simulink model "h2_containment_static_3d"  (R2022b)
settings: Solver=FixedStepAuto  StartTime=0.0  StopTime=15  FixedStep=0.01  RelTol=1e-3
values from neighbouring files (symbols this model uses):
  A = [0, 0,-1 ;0 0 2; 1 0  -1.5]    [containment_staic_3d.m]    (also in containment_staic_3d_paper.m)
  Af = kron(IM,A)    [containment_staic_3d.m]    (also in containment_staic_3d_paper.m)
  Al = kron(Inm,A)    [containment_staic_3d.m]    (also in containment_staic_3d_paper.m)
  Bf = kron(IM,B)    [containment_staic_3d.m]    (also in containment_staic_3d_paper.m)
  Cd = kron(IM,C)+kron(L1,D*K)    [containment_staic_3d.m]    (also in containment_staic_3d_paper.m)
  Ef = kron(IM,E)    [containment_staic_3d.m]    (also in containment_staic_3d_paper.m)
  Kk = kron(IM,K)    [containment_staic_3d.m]    (also in containment_staic_3d_paper.m)
  Lk1 = kron(L1,eye(3))    [containment_staic_3d.m]    (also in containment_staic_3d_paper.m)
  Lk2 = kron(L2,eye(3))    [containment_staic_3d.m]    (also in containment_staic_3d_paper.m)
  xf = xint(1:18)'    [containment_staic_3d.m]    (also in containment_staic_3d_paper.m)
  Xint = kron(L1,eye(3))*xf+kron(L2,eye(3))*xl    [containment_staic_3d.m]    (also in containment_staic_3d_paper.m)
  xl = xint(19:27)'    [containment_staic_3d.m]    (also in containment_staic_3d_paper.m)
settings Model: Creator=lenovo  LastModifiedBy=herrg
settings SolverCC: AlgebraicLoopSolver=TrustRegion
settings DebuggingCC: UnconnectedInputMsg=warning  UnconnectedOutputMsg=warning  UnconnectedLineMsg=warning  SFMachineParentedDataDiag=warning
settings ModelReferenceCC: EnableRefExpFcnMdlSchedulingChecks=on
settings RTWCC: DLArmComputeVersion=19.05

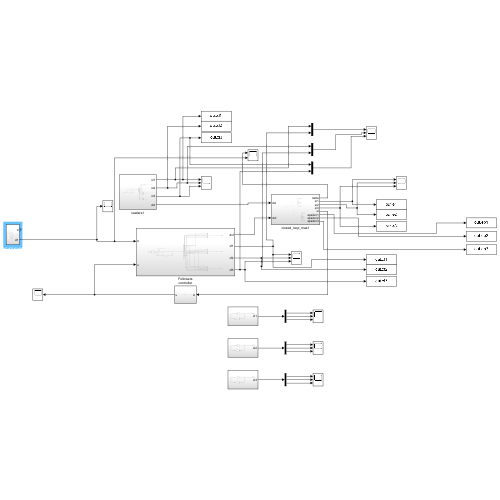
[thumbnail: Simulink's stored preview of the top-level diagram]
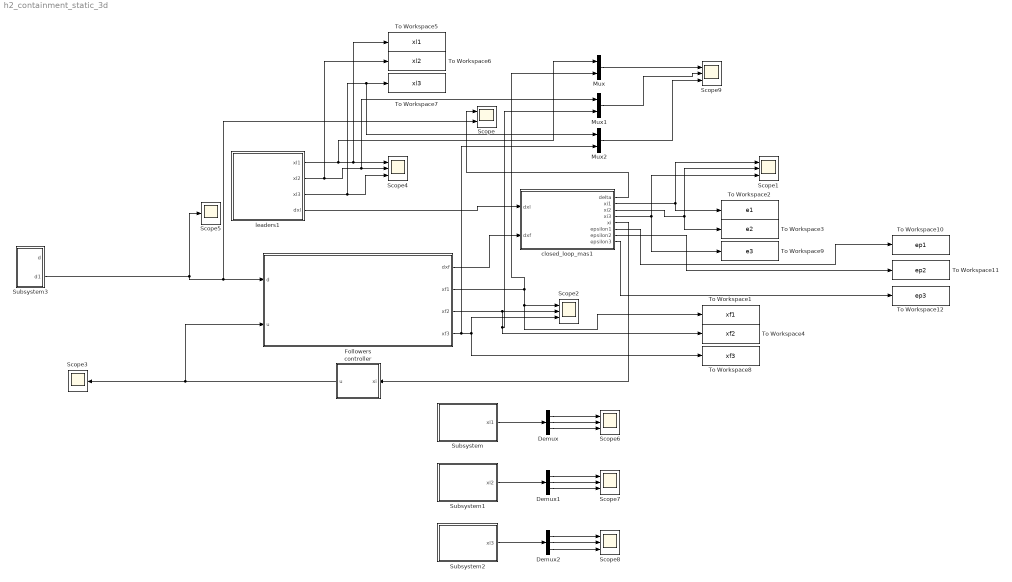
== system h2_containment_static_3d ==
  Demux : Demux  Outputs=3
  Demux1 : Demux  Outputs=3
  Demux2 : Demux  Outputs=3
  Followers : Subsystem
  Mux : Mux  Inputs=2
  Mux1 : Mux  Inputs=2
  Mux2 : Mux  Inputs=2
  Scope : Scope  NumInputPorts=2
  Scope{1..2,4,6..9} (7 alike) : Scope  NumInputPorts=3
  Scope3 : Scope
  Scope5 : Scope
  Subsystem : Subsystem
  Subsystem1 : Subsystem
  Subsystem2 : Subsystem
  Subsystem3 : Subsystem
  To Workspace1 : ToWorkspace  VariableName=xf1  SampleTime=-1
  To Workspace10 : ToWorkspace  VariableName=ep1  SampleTime=-1
  To Workspace11 : ToWorkspace  VariableName=ep2  SampleTime=-1
  To Workspace12 : ToWorkspace  VariableName=ep3  SampleTime=-1
  To Workspace2 : ToWorkspace  VariableName=e1  SampleTime=-1
  To Workspace3 : ToWorkspace  VariableName=e2  SampleTime=-1
  To Workspace4 : ToWorkspace  VariableName=xf2  SampleTime=-1
  To Workspace5 : ToWorkspace  VariableName=xl1  SampleTime=-1
  To Workspace6 : ToWorkspace  VariableName=xl2  SampleTime=-1
  To Workspace7 : ToWorkspace  VariableName=xl3  SampleTime=-1
  To Workspace8 : ToWorkspace  VariableName=xf3  SampleTime=-1
  To Workspace9 : ToWorkspace  VariableName=e3  SampleTime=-1
  closed_loop_mas1 : Subsystem
  controller : Subsystem
  leaders1 : Subsystem
  wires:
  leaders1/2(xl2) -> Scope4/2, Mux1/1, To Workspace6/1
  closed_loop_mas1/1(delta) -> Scope/1
  Followers/3(xf2) -> Scope2/2, Mux1/2, To Workspace4/1
  Followers/2(xf1) -> To Workspace1/1, Scope2/1, Mux/2
  closed_loop_mas1/5(xi) -> controller/1(xi)
  closed_loop_mas1/3(xi2) -> Scope1/2, To Workspace3/1
  closed_loop_mas1/2(xi1) -> To Workspace2/1, Scope1/1
  Demux1/1 -> Scope7/1
  Subsystem1/1(xl2) -> Demux1/1
  Demux1/2 -> Scope7/2
  leaders1/4(dxl) -> closed_loop_mas1/1(dxl)
  Followers/1(dxf) -> closed_loop_mas1/2(dxf)
  controller/1(u) -> Followers/2(u), Scope3/1
  Demux/2 -> Scope6/2
  Mux1/1 -> Scope9/2
  leaders1/1(xl1) -> Mux/1, To Workspace5/1, Scope4/1
  Demux/1 -> Scope6/1
  Mux/1 -> Scope9/1
  Demux2/2 -> Scope8/2
  Demux2/1 -> Scope8/1
  Subsystem/1(xl1) -> Demux/1
  Subsystem2/1(xl3) -> Demux2/1
  Demux/3 -> Scope6/3
  Demux1/3 -> Scope7/3
  Demux2/3 -> Scope8/3
  leaders1/3(xl3) -> Mux2/1, To Workspace7/1, Scope4/3
  Followers/4(xf3) -> Mux2/2, To Workspace8/1, Scope2/3
  closed_loop_mas1/4(xi3) -> To Workspace9/1, Scope1/3
  Mux2/1 -> Scope9/3
  closed_loop_mas1/6(epsilon1) -> To Workspace10/1
  closed_loop_mas1/7(epsilon2) -> To Workspace11/1
  closed_loop_mas1/8(epsilon3) -> To Workspace12/1
  Subsystem3/2(d1) -> Scope5/1, Scope/2, Followers/1(d)

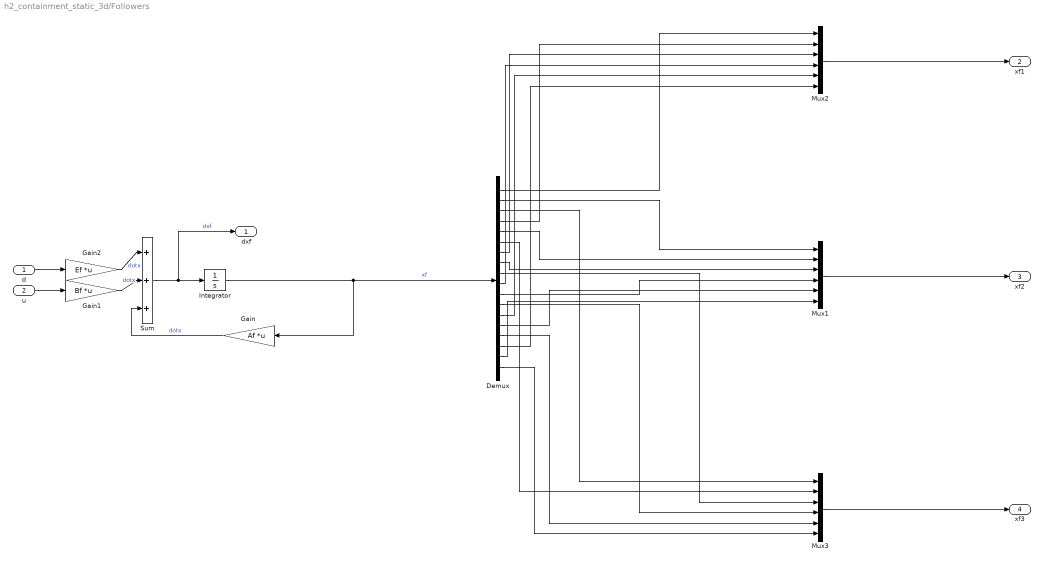
== system h2_containment_static_3d/Followers ==
  d : Inport
  u : Inport  Port=2
  Demux : Demux  Outputs=18
  Gain : Gain  Gain=Af  Multiplication=Matrix(K*u) (u vector)
  Gain1 : Gain  Gain=Bf  Multiplication=Matrix(K*u) (u vector)
  Gain2 : Gain  Gain=Ef  Multiplication=Matrix(K*u) (u vector)
  Integrator : Integrator  InitialCondition=xf
  Mux1 : Mux  Inputs=6
  Mux2 : Mux  Inputs=6
  Mux3 : Mux  Inputs=6
  Sum : Sum  Inputs=|+++
  dxf : Outport
  xf1 : Outport  Port=2
  xf2 : Outport  Port=3
  xf3 : Outport  Port=4
  wires:
  Gain/1 -> Sum/3  "dotx"
  u/1 -> Gain1/1
  d/1 -> Gain2/1
  Gain1/1 -> Sum/2  "dotx"
  Gain2/1 -> Sum/1  "dotx"
  Sum/1 -> dxf/1, Integrator/1  "dxf"
  Integrator/1 -> Gain/1, Demux/1  "xf"
  Mux2/1 -> xf1/1
  Mux1/1 -> xf2/1
  Mux3/1 -> xf3/1
  Demux/1 -> Mux2/1
  Demux/2 -> Mux1/1
  Demux/3 -> Mux3/1
  Demux/4 -> Mux2/2
  Demux/5 -> Mux1/2
  Demux/6 -> Mux3/2
  Demux/7 -> Mux2/3
  Demux/8 -> Mux1/3
  Demux/9 -> Mux3/3
  Demux/10 -> Mux2/4
  Demux/11 -> Mux1/4
  Demux/12 -> Mux3/4
  Demux/13 -> Mux2/5
  Demux/14 -> Mux1/5
  Demux/15 -> Mux3/5
  Demux/16 -> Mux2/6
  Demux/17 -> Mux1/6
  Demux/18 -> Mux3/6

== system h2_containment_static_3d/Subsystem ==
  Gain2 : Gain  Gain=A  Multiplication=Matrix(K*u) (u vector)
  Integrator : Integrator  InitialCondition=xl(1:3)
  xl1 : Outport
  wires:
  Integrator/1 -> xl1/1, Gain2/1  "x"
  Gain2/1 -> Integrator/1  "dotx"

== system h2_containment_static_3d/Subsystem1 ==
  Gain2 : Gain  Gain=A  Multiplication=Matrix(K*u) (u vector)
  Integrator : Integrator  InitialCondition=xl(4:6)
  xl2 : Outport
  wires:
  Integrator/1 -> xl2/1, Gain2/1  "x"
  Gain2/1 -> Integrator/1  "dotx"

== system h2_containment_static_3d/Subsystem2 ==
  Gain2 : Gain  Gain=A  Multiplication=Matrix(K*u) (u vector)
  Integrator : Integrator  InitialCondition=xl(7:9)
  xl3 : Outport
  wires:
  Integrator/1 -> xl3/1, Gain2/1  "x"
  Gain2/1 -> Integrator/1  "dotx"

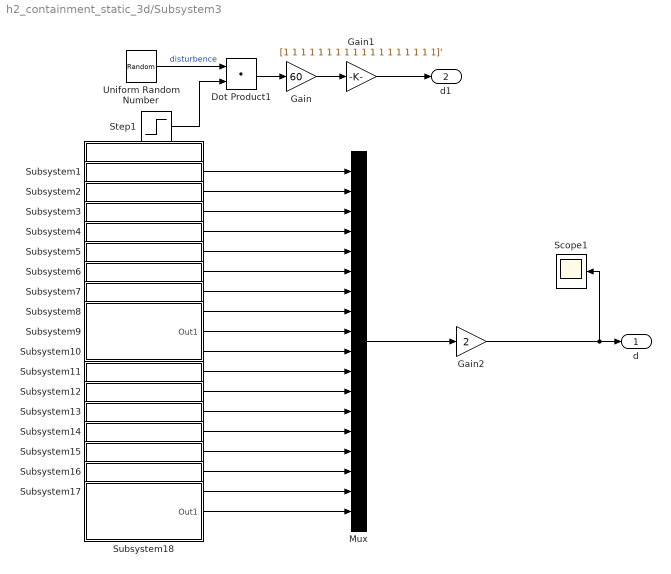
== system h2_containment_static_3d/Subsystem3 ==
  Dot Product1 : DotProduct  OutDataTypeStr=Inherit: Inherit via internal rule
  Gain : Gain  Gain=60
  Gain1 : Gain  Gain=[1 1 1 1 1 1 1 1 1 1 1 1 1 1 1 1 1 1]'
  Gain2 : Gain  Gain=2
  Mux : Mux  Inputs=18
  Scope1 : Scope
  Step1 : Step  Time=1000  Before=1  After=0  SampleTime=0
  Subsystem1 : Subsystem
  Subsystem10 : Subsystem
  Subsystem11 : Subsystem
  Subsystem12 : Subsystem
  Subsystem13 : Subsystem
  Subsystem14 : Subsystem
  Subsystem15 : Subsystem
  Subsystem16 : Subsystem
  Subsystem17 : Subsystem
  Subsystem18 : Subsystem
  Subsystem2 : Subsystem
  Subsystem3 : Subsystem
  Subsystem4 : Subsystem
  Subsystem5 : Subsystem
  Subsystem6 : Subsystem
  Subsystem7 : Subsystem
  Subsystem8 : Subsystem
  Subsystem9 : Subsystem
  Uniform Random Number : UniformRandomNumber  SampleTime=0.1
  d : Outport
  d1 : Outport  Port=2
  wires:
  Gain1/1 -> d1/1
  Gain/1 -> Gain1/1
  Step1/1 -> Dot Product1/2
  Dot Product1/1 -> Gain/1
  Uniform Random Number/1 -> Dot Product1/1  "disturbence"
  Subsystem13/1(Out1) -> Mux/13
  Subsystem11/1(Out1) -> Mux/11
  Subsystem18/1(Out1) -> Mux/18
  Mux/1 -> Gain2/1
  Subsystem9/1(Out1) -> Mux/9
  Subsystem10/1(Out1) -> Mux/10
  Subsystem8/1(Out1) -> Mux/8
  Subsystem15/1(Out1) -> Mux/15
  Subsystem7/1(Out1) -> Mux/7
  Subsystem14/1(Out1) -> Mux/14
  Subsystem17/1(Out1) -> Mux/17
  Subsystem16/1(Out1) -> Mux/16
  Subsystem4/1(Out1) -> Mux/4
  Subsystem3/1(Out1) -> Mux/3
  Subsystem1/1(Out1) -> Mux/1
  Subsystem2/1(Out1) -> Mux/2
  Subsystem12/1(Out1) -> Mux/12
  Subsystem6/1(Out1) -> Mux/6
  Subsystem5/1(Out1) -> Mux/5
  Gain2/1 -> Scope1/1, d/1

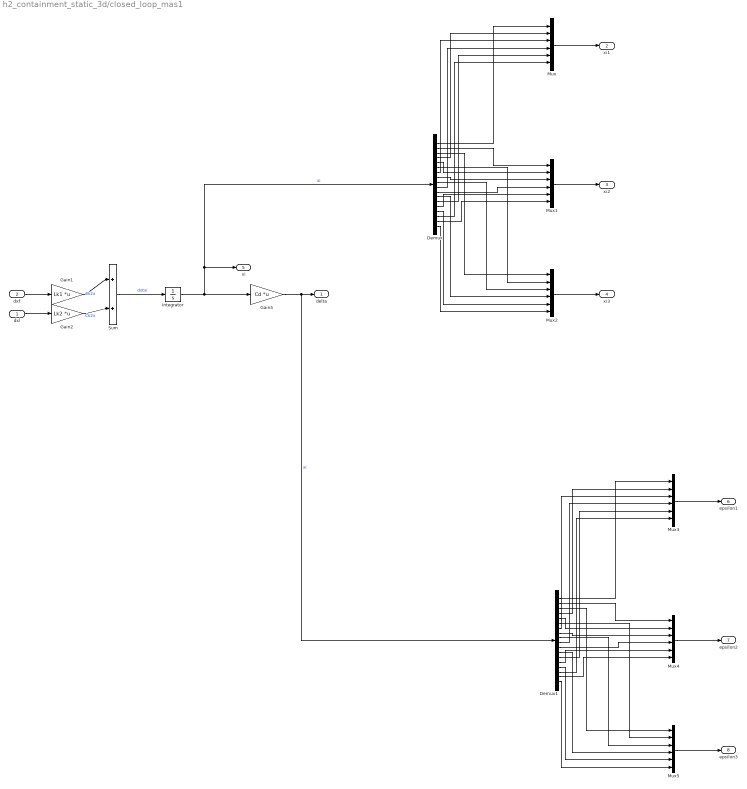
== system h2_containment_static_3d/closed_loop_mas1 ==
  dxl : Inport
  dxf : Inport  Port=2
  Demux : Demux  Outputs=18
  Demux1 : Demux  Outputs=18
  Gain1 : Gain  Gain=Lk1  Multiplication=Matrix(K*u) (u vector)
  Gain2 : Gain  Gain=Lk2  Multiplication=Matrix(K*u) (u vector)
  Gain5 : Gain  Gain=Cd  Multiplication=Matrix(K*u) (u vector)
  Integrator : Integrator  InitialCondition=Xint
  Mux{,1..5} (6 alike) : Mux  Inputs=6
  Sum : Sum  Inputs=|++
  delta : Outport
  xi1 : Outport  Port=2
  xi2 : Outport  Port=3
  xi3 : Outport  Port=4
  xi : Outport  Port=5
  epsilon1 : Outport  Port=6
  epsilon2 : Outport  Port=7
  epsilon3 : Outport  Port=8
  wires:
  Integrator/1 -> Demux/1, xi/1, Gain5/1  "xi"
  Sum/1 -> Integrator/1  "dotxi"
  Mux/1 -> xi1/1
  Mux1/1 -> xi2/1
  dxf/1 -> Gain1/1
  dxl/1 -> Gain2/1
  Gain1/1 -> Sum/1  "Ck2x"
  Gain2/1 -> Sum/2  "Ck2x"
  Mux2/1 -> xi3/1
  Demux/1 -> Mux/1
  Demux/2 -> Mux1/1
  Demux/3 -> Mux2/1
  Demux/4 -> Mux/2
  Demux/5 -> Mux1/2
  Demux/6 -> Mux2/2
  Demux/7 -> Mux/3
  Demux/8 -> Mux1/3
  Demux/9 -> Mux2/3
  Demux/10 -> Mux/4
  Demux/11 -> Mux1/4
  Demux/12 -> Mux2/4
  Demux/13 -> Mux/5
  Demux/14 -> Mux1/5
  Demux/15 -> Mux2/5
  Demux/16 -> Mux/6
  Demux/17 -> Mux1/6
  Demux/18 -> Mux2/6
  Demux1/16 -> Mux3/6
  Demux1/17 -> Mux4/6
  Demux1/4 -> Mux3/2
  Demux1/15 -> Mux5/5
  Demux1/10 -> Mux3/4
  Demux1/14 -> Mux4/5
  Demux1/11 -> Mux4/4
  Demux1/5 -> Mux4/2
  Demux1/7 -> Mux3/3
  Demux1/9 -> Mux5/3
  Demux1/18 -> Mux5/6
  Demux1/13 -> Mux3/5
  Demux1/12 -> Mux5/4
  Demux1/6 -> Mux5/2
  Mux5/1 -> epsilon3/1
  Demux1/2 -> Mux4/1
  Demux1/1 -> Mux3/1
  Demux1/3 -> Mux5/1
  Mux4/1 -> epsilon2/1
  Gain5/1 -> Demux1/1, delta/1  "xi"
  Demux1/8 -> Mux4/3
  Mux3/1 -> epsilon1/1

== system h2_containment_static_3d/controller ==
  xi : Inport
  Gain2 : Gain  Gain=Kk  Multiplication=Matrix(K*u) (u vector)
  u : Outport
  wires:
  Gain2/1 -> u/1
  xi/1 -> Gain2/1

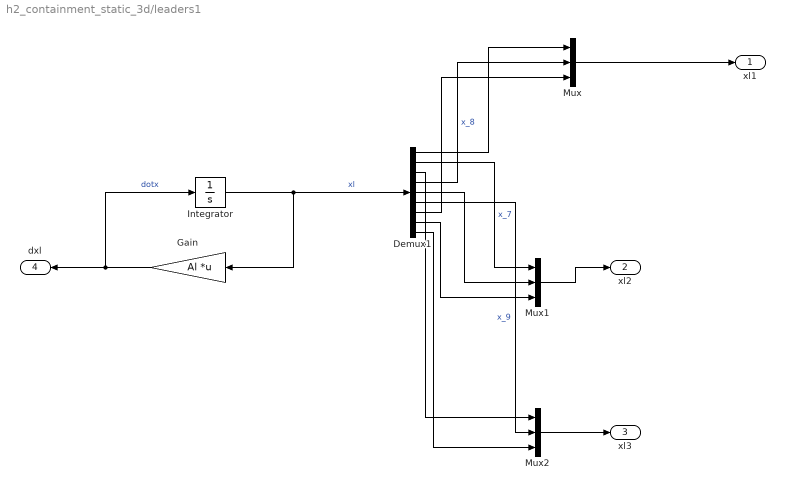
== system h2_containment_static_3d/leaders1 ==
  Demux1 : Demux  Outputs=9
  Gain : Gain  Gain=Al  Multiplication=Matrix(K*u) (u vector)
  Integrator : Integrator  InitialCondition=xl
  Mux : Mux  Inputs=3
  Mux1 : Mux  Inputs=3
  Mux2 : Mux  Inputs=3
  xl1 : Outport
  xl2 : Outport  Port=2
  xl3 : Outport  Port=3
  dxl : Outport  Port=4
  wires:
  Gain/1 -> dxl/1, Integrator/1  "dotx"
  Integrator/1 -> Gain/1, Demux1/1  "xl"
  Mux1/1 -> xl2/1
  Mux/1 -> xl1/1
  Demux1/1 -> Mux/1
  Demux1/4 -> Mux/2  "x_8"
  Demux1/7 -> Mux/3
  Demux1/2 -> Mux1/1  "x_7"
  Demux1/5 -> Mux1/2
  Demux1/8 -> Mux1/3
  Mux2/1 -> xl3/1
  Demux1/3 -> Mux2/1
  Demux1/6 -> Mux2/2  "x_9"
  Demux1/9 -> Mux2/3

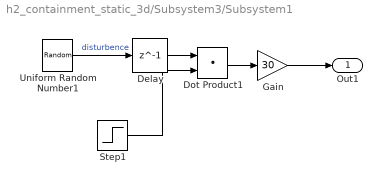
== system h2_containment_static_3d/Subsystem3/Subsystem1 ==
  Delay : Delay  DelayLength=1  SampleTime=0.01
  Dot Product1 : DotProduct  OutDataTypeStr=Inherit: Inherit via internal rule
  Gain : Gain  Gain=30
  Step1 : Step  Time=999  Before=1  After=0  SampleTime=0
  Uniform Random Number1 : UniformRandomNumber  SampleTime=0.1
  Out1 : Outport
  wires:
  Uniform Random Number1/1 -> Delay/1  "disturbence"
  Gain/1 -> Out1/1
  Dot Product1/1 -> Gain/1
  Step1/1 -> Dot Product1/2
  Delay/1 -> Dot Product1/1

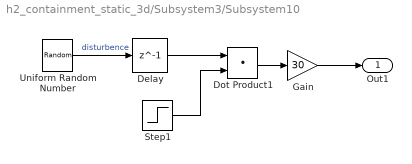
== system h2_containment_static_3d/Subsystem3/Subsystem10 ==
  Delay : Delay  DelayLength=1  SampleTime=0.01
  Dot Product1 : DotProduct  OutDataTypeStr=Inherit: Inherit via internal rule
  Gain : Gain  Gain=30
  Step1 : Step  Time=1000  Before=1  After=0  SampleTime=0
  Uniform Random Number : UniformRandomNumber  SampleTime=0.1
  Out1 : Outport
  wires:
  Uniform Random Number/1 -> Delay/1  "disturbence"
  Step1/1 -> Dot Product1/2
  Gain/1 -> Out1/1
  Dot Product1/1 -> Gain/1
  Delay/1 -> Dot Product1/1

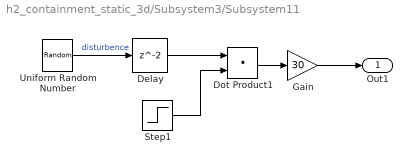
== system h2_containment_static_3d/Subsystem3/Subsystem11 ==
  Delay : Delay  SampleTime=0.01
  Dot Product1 : DotProduct  OutDataTypeStr=Inherit: Inherit via internal rule
  Gain : Gain  Gain=30
  Step1 : Step  Time=1000  Before=1  After=0  SampleTime=0
  Uniform Random Number : UniformRandomNumber  SampleTime=0.1
  Out1 : Outport
  wires:
  Uniform Random Number/1 -> Delay/1  "disturbence"
  Step1/1 -> Dot Product1/2
  Gain/1 -> Out1/1
  Dot Product1/1 -> Gain/1
  Delay/1 -> Dot Product1/1

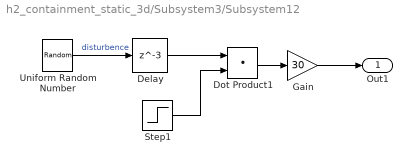
== system h2_containment_static_3d/Subsystem3/Subsystem12 ==
  Delay : Delay  DelayLength=3  SampleTime=0.01
  Dot Product1 : DotProduct  OutDataTypeStr=Inherit: Inherit via internal rule
  Gain : Gain  Gain=30
  Step1 : Step  Time=1000  Before=1  After=0  SampleTime=0
  Uniform Random Number : UniformRandomNumber  SampleTime=0.1
  Out1 : Outport
  wires:
  Uniform Random Number/1 -> Delay/1  "disturbence"
  Step1/1 -> Dot Product1/2
  Gain/1 -> Out1/1
  Dot Product1/1 -> Gain/1
  Delay/1 -> Dot Product1/1

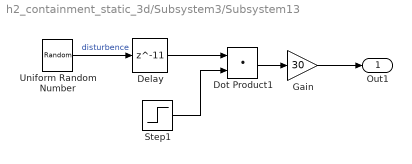
== system h2_containment_static_3d/Subsystem3/Subsystem13 ==
  Delay : Delay  DelayLength=11  SampleTime=0.01
  Dot Product1 : DotProduct  OutDataTypeStr=Inherit: Inherit via internal rule
  Gain : Gain  Gain=30
  Step1 : Step  Time=1000  Before=1  After=0  SampleTime=0
  Uniform Random Number : UniformRandomNumber  SampleTime=0.1
  Out1 : Outport
  wires:
  Uniform Random Number/1 -> Delay/1  "disturbence"
  Step1/1 -> Dot Product1/2
  Gain/1 -> Out1/1
  Dot Product1/1 -> Gain/1
  Delay/1 -> Dot Product1/1

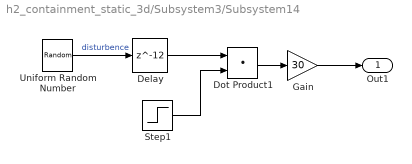
== system h2_containment_static_3d/Subsystem3/Subsystem14 ==
  Delay : Delay  DelayLength=12  SampleTime=0.01
  Dot Product1 : DotProduct  OutDataTypeStr=Inherit: Inherit via internal rule
  Gain : Gain  Gain=30
  Step1 : Step  Time=1000  Before=1  After=0  SampleTime=0
  Uniform Random Number : UniformRandomNumber  SampleTime=0.1
  Out1 : Outport
  wires:
  Uniform Random Number/1 -> Delay/1  "disturbence"
  Step1/1 -> Dot Product1/2
  Gain/1 -> Out1/1
  Dot Product1/1 -> Gain/1
  Delay/1 -> Dot Product1/1

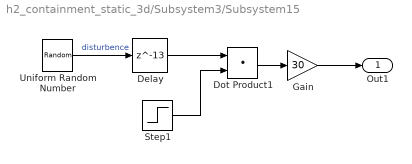
== system h2_containment_static_3d/Subsystem3/Subsystem15 ==
  Delay : Delay  DelayLength=13  SampleTime=0.01
  Dot Product1 : DotProduct  OutDataTypeStr=Inherit: Inherit via internal rule
  Gain : Gain  Gain=30
  Step1 : Step  Time=1000  Before=1  After=0  SampleTime=0
  Uniform Random Number : UniformRandomNumber  SampleTime=0.1
  Out1 : Outport
  wires:
  Uniform Random Number/1 -> Delay/1  "disturbence"
  Step1/1 -> Dot Product1/2
  Gain/1 -> Out1/1
  Dot Product1/1 -> Gain/1
  Delay/1 -> Dot Product1/1

== system h2_containment_static_3d/Subsystem3/Subsystem16 ==
  Delay : Delay  DelayLength=14  SampleTime=0.01
  Dot Product1 : DotProduct  OutDataTypeStr=Inherit: Inherit via internal rule
  Gain : Gain  Gain=30
  Step1 : Step  Time=1000  Before=1  After=0  SampleTime=0
  Uniform Random Number : UniformRandomNumber  SampleTime=0.1
  Out1 : Outport
  wires:
  Uniform Random Number/1 -> Delay/1  "disturbence"
  Step1/1 -> Dot Product1/2
  Gain/1 -> Out1/1
  Dot Product1/1 -> Gain/1
  Delay/1 -> Dot Product1/1

== system h2_containment_static_3d/Subsystem3/Subsystem17 ==
  Delay : Delay  DelayLength=15  SampleTime=0.01
  Dot Product1 : DotProduct  OutDataTypeStr=Inherit: Inherit via internal rule
  Gain : Gain  Gain=30
  Step1 : Step  Time=1000  Before=1  After=0  SampleTime=0
  Uniform Random Number : UniformRandomNumber  SampleTime=0.1
  Out1 : Outport
  wires:
  Uniform Random Number/1 -> Delay/1  "disturbence"
  Step1/1 -> Dot Product1/2
  Gain/1 -> Out1/1
  Dot Product1/1 -> Gain/1
  Delay/1 -> Dot Product1/1

== system h2_containment_static_3d/Subsystem3/Subsystem18 ==
  Delay : Delay  DelayLength=16  SampleTime=0.01
  Dot Product1 : DotProduct  OutDataTypeStr=Inherit: Inherit via internal rule
  Gain : Gain  Gain=30
  Step1 : Step  Time=1000  Before=1  After=0  SampleTime=0
  Uniform Random Number : UniformRandomNumber  SampleTime=0.1
  Out1 : Outport
  wires:
  Uniform Random Number/1 -> Delay/1  "disturbence"
  Step1/1 -> Dot Product1/2
  Gain/1 -> Out1/1
  Dot Product1/1 -> Gain/1
  Delay/1 -> Dot Product1/1

== system h2_containment_static_3d/Subsystem3/Subsystem2 ==
  Delay : Delay  SampleTime=0.01
  Dot Product1 : DotProduct  OutDataTypeStr=Inherit: Inherit via internal rule
  Gain : Gain  Gain=30
  Step1 : Step  Time=1000  Before=1  After=0  SampleTime=0
  Uniform Random Number : UniformRandomNumber  SampleTime=0.1
  Out1 : Outport
  wires:
  Uniform Random Number/1 -> Delay/1  "disturbence"
  Step1/1 -> Dot Product1/2
  Gain/1 -> Out1/1
  Dot Product1/1 -> Gain/1
  Delay/1 -> Dot Product1/1

== system h2_containment_static_3d/Subsystem3/Subsystem3 ==
  Delay : Delay  DelayLength=3  SampleTime=0.01
  Dot Product1 : DotProduct  OutDataTypeStr=Inherit: Inherit via internal rule
  Gain : Gain  Gain=30
  Step1 : Step  Time=1000  Before=1  After=0  SampleTime=0
  Uniform Random Number : UniformRandomNumber  SampleTime=0.1
  Out1 : Outport
  wires:
  Uniform Random Number/1 -> Delay/1  "disturbence"
  Step1/1 -> Dot Product1/2
  Gain/1 -> Out1/1
  Dot Product1/1 -> Gain/1
  Delay/1 -> Dot Product1/1

== system h2_containment_static_3d/Subsystem3/Subsystem4 ==
  Delay : Delay  DelayLength=4  SampleTime=0.01
  Dot Product1 : DotProduct  OutDataTypeStr=Inherit: Inherit via internal rule
  Gain : Gain  Gain=30
  Step1 : Step  Time=1000  Before=1  After=0  SampleTime=0
  Uniform Random Number : UniformRandomNumber  SampleTime=0.1
  Out1 : Outport
  wires:
  Uniform Random Number/1 -> Delay/1  "disturbence"
  Step1/1 -> Dot Product1/2
  Gain/1 -> Out1/1
  Dot Product1/1 -> Gain/1
  Delay/1 -> Dot Product1/1

== system h2_containment_static_3d/Subsystem3/Subsystem5 ==
  Delay : Delay  DelayLength=5  SampleTime=0.01
  Dot Product1 : DotProduct  OutDataTypeStr=Inherit: Inherit via internal rule
  Gain : Gain  Gain=30
  Step1 : Step  Time=1000  Before=1  After=0  SampleTime=0
  Uniform Random Number : UniformRandomNumber  SampleTime=0.1
  Out1 : Outport
  wires:
  Uniform Random Number/1 -> Delay/1  "disturbence"
  Step1/1 -> Dot Product1/2
  Gain/1 -> Out1/1
  Dot Product1/1 -> Gain/1
  Delay/1 -> Dot Product1/1

== system h2_containment_static_3d/Subsystem3/Subsystem6 ==
  Delay : Delay  DelayLength=6  SampleTime=0.01
  Dot Product1 : DotProduct  OutDataTypeStr=Inherit: Inherit via internal rule
  Gain : Gain  Gain=30
  Step1 : Step  Time=1000  Before=1  After=0  SampleTime=0
  Uniform Random Number : UniformRandomNumber  SampleTime=0.1
  Out1 : Outport
  wires:
  Uniform Random Number/1 -> Delay/1  "disturbence"
  Step1/1 -> Dot Product1/2
  Gain/1 -> Out1/1
  Dot Product1/1 -> Gain/1
  Delay/1 -> Dot Product1/1

== system h2_containment_static_3d/Subsystem3/Subsystem7 ==
  Delay : Delay  DelayLength=7  SampleTime=0.01
  Dot Product1 : DotProduct  OutDataTypeStr=Inherit: Inherit via internal rule
  Gain : Gain  Gain=30
  Step1 : Step  Time=1000  Before=1  After=0  SampleTime=0
  Uniform Random Number : UniformRandomNumber  SampleTime=0.1
  Out1 : Outport
  wires:
  Uniform Random Number/1 -> Delay/1  "disturbence"
  Step1/1 -> Dot Product1/2
  Gain/1 -> Out1/1
  Dot Product1/1 -> Gain/1
  Delay/1 -> Dot Product1/1

== system h2_containment_static_3d/Subsystem3/Subsystem8 ==
  Delay : Delay  DelayLength=8  SampleTime=0.01
  Dot Product1 : DotProduct  OutDataTypeStr=Inherit: Inherit via internal rule
  Gain : Gain  Gain=30
  Step1 : Step  Time=1000  Before=1  After=0  SampleTime=0
  Uniform Random Number : UniformRandomNumber  SampleTime=0.1
  Out1 : Outport
  wires:
  Uniform Random Number/1 -> Delay/1  "disturbence"
  Step1/1 -> Dot Product1/2
  Gain/1 -> Out1/1
  Dot Product1/1 -> Gain/1
  Delay/1 -> Dot Product1/1

== system h2_containment_static_3d/Subsystem3/Subsystem9 ==
  Delay : Delay  DelayLength=9  SampleTime=0.01
  Dot Product1 : DotProduct  OutDataTypeStr=Inherit: Inherit via internal rule
  Gain : Gain  Gain=30
  Step1 : Step  Time=1000  Before=1  After=0  SampleTime=0
  Uniform Random Number : UniformRandomNumber  SampleTime=0.1
  Out1 : Outport
  wires:
  Uniform Random Number/1 -> Delay/1  "disturbence"
  Step1/1 -> Dot Product1/2
  Gain/1 -> Out1/1
  Dot Product1/1 -> Gain/1
  Delay/1 -> Dot Product1/1
